simulink model "pd_path_sg"  (R2013b)
settings: Solver=ode45  StartTime=0.0  StopTime=10  RelTol=1e-3
undefined symbols (not defined in the file or in its folder): A, A2, B, C, D, EVAL, i, output_samp_bcoef, PCIN, reg_pk_lim, reg_plim, reg_scale, reg_sr_lim, reg_staclr, reg_txgain, THIS_DATE, W, X, Z
undefined symbols (not defined in the file): lut_address, lut_address_s5, reg_dltap
libraries: xbsIndex_r4 x3819, lut_ram_vhdl x32
(part 2 of 31)

== system pd_path_sg/gmp_model_A ==
  chi : Inport
  x : Inport  Port=2
  c : Inport  Port=3
  Delay1 : xbsIndex_r4/Delay  rst=off  infoeditControl=Selection of Reset will increase slice count due to use of real FFs and instead of SRLs  en=off  latency=1  reg_retiming=off  dbl_ovrd=off  block_type=delay
      settings: infoedit=Hardware notes: A delay line is a chain, each link of which is an SRL16 or SRL32 followed by a flip-flop.
  Delay2 : xbsIndex_r4/Delay  rst=off  infoeditControl=Selection of Reset will increase slice count due to use of real FFs and instead of SRLs  en=off  latency=1  reg_retiming=off  dbl_ovrd=off  block_type=delay
      settings: infoedit=Hardware notes: A delay line is a chain, each link of which is an SRL16 or SRL32 followed by a flip-flop.
  Delay3 : xbsIndex_r4/Delay  rst=off  infoeditControl=Selection of Reset will increase slice count due to use of real FFs and instead of SRLs  en=off  latency=1  reg_retiming=off  dbl_ovrd=off  block_type=delay
      settings: infoedit=Hardware notes: A delay line is a chain, each link of which is an SRL16 or SRL32 followed by a flip-flop.
  Demux : Demux  Outputs=7
  Demux1 : Demux  Outputs=7
  Mux : Mux  Inputs=2
  bit_cut : Subsystem  mask{cut=12, left=17}
  bit_cut1 : Subsystem  mask{cut=12, left=17}
  cmp_mul 0 : Subsystem
  cmp_mul1 : Subsystem
  cmp_mul2 : Subsystem
  cmp_mul3 : Subsystem
  cmp_mul4 : Subsystem
  cmp_mul5 : Subsystem
  cmp_mul6 : Subsystem
  cho : Outport
  y : Outport  Port=2
  wires:
  Demux/1 -> [x0]
  cmp_mul 0/3(pcout_i) -> cmp_mul1/3(pcin_i)
  Mux/1 -> y/1
  x/1 -> Demux/1
  c/1 -> Demux1/1
  cmp_mul 0/4(pcout_q) -> cmp_mul1/4(pcin_q)
  [x0] -> cmp_mul 0/1(x)
  Demux/2 -> [x1]
  [x1] -> cmp_mul1/1(x)
  Demux/3 -> [x2]
  [x2] -> cmp_mul2/1(x)
  Demux/4 -> [x3]
  Demux/5 -> [x4]
  Demux/6 -> [x5]
  Demux/7 -> [x6]
  Demux1/1 -> [c0]
  [c0] -> cmp_mul 0/2(coef)
  [c1] -> cmp_mul1/2(coef)
  Demux1/2 -> [c1]
  [c2] -> cmp_mul2/2(coef)
  Demux1/3 -> [c2]
  Demux1/4 -> [c3]
  Demux1/5 -> [c4]
  Demux1/6 -> [c5]
  Demux1/7 -> [c6]
  Delay1/1 -> Mux/1
  Delay2/1 -> Mux/2
  bit_cut/1(q) -> Delay1/1
  bit_cut1/1(q) -> Delay2/1
  cmp_mul1/3(pcout_i) -> cmp_mul2/3(pcin_i)
  cmp_mul1/4(pcout_q) -> cmp_mul2/4(pcin_q)
  cmp_mul2/3(pcout_i) -> cmp_mul3/3(pcin_i)
  cmp_mul2/4(pcout_q) -> cmp_mul3/4(pcin_q)
  [x3] -> cmp_mul3/1(x)
  [c3] -> cmp_mul3/2(coef)
  cmp_mul3/3(pcout_i) -> cmp_mul4/3(pcin_i)
  cmp_mul3/4(pcout_q) -> cmp_mul4/4(pcin_q)
  [c4] -> cmp_mul4/2(coef)
  [x4] -> cmp_mul4/1(x)
  cmp_mul4/3(pcout_i) -> cmp_mul5/3(pcin_i)
  cmp_mul4/4(pcout_q) -> cmp_mul5/4(pcin_q)
  [c5] -> cmp_mul5/2(coef)
  [x5] -> cmp_mul5/1(x)
  cmp_mul5/3(pcout_i) -> cmp_mul6/3(pcin_i)
  cmp_mul5/4(pcout_q) -> cmp_mul6/4(pcin_q)
  [x6] -> cmp_mul6/1(x)
  [c6] -> cmp_mul6/2(coef)
  cmp_mul6/3(iout) -> bit_cut/1(d)
  cmp_mul6/4(qout) -> bit_cut1/1(d)
  chi/1 -> Delay3/1
  Delay3/1 -> cho/1

== system pd_path_sg/gmp_model_B ==
  chi : Inport
  x : Inport  Port=2
  c : Inport  Port=3
  Delay1 : xbsIndex_r4/Delay  rst=off  infoeditControl=Selection of Reset will increase slice count due to use of real FFs and instead of SRLs  en=off  latency=1  reg_retiming=off  dbl_ovrd=off  block_type=delay
      settings: infoedit=Hardware notes: A delay line is a chain, each link of which is an SRL16 or SRL32 followed by a flip-flop.
  Delay2 : xbsIndex_r4/Delay  rst=off  infoeditControl=Selection of Reset will increase slice count due to use of real FFs and instead of SRLs  en=off  latency=1  reg_retiming=off  dbl_ovrd=off  block_type=delay
      settings: infoedit=Hardware notes: A delay line is a chain, each link of which is an SRL16 or SRL32 followed by a flip-flop.
  Delay3 : xbsIndex_r4/Delay  rst=off  infoeditControl=Selection of Reset will increase slice count due to use of real FFs and instead of SRLs  en=off  latency=1  reg_retiming=off  dbl_ovrd=off  block_type=delay
      settings: infoedit=Hardware notes: A delay line is a chain, each link of which is an SRL16 or SRL32 followed by a flip-flop.
  Demux : Demux  Outputs=7
  Demux1 : Demux  Outputs=7
  Mux : Mux  Inputs=2
  bit_cut : Subsystem  mask{cut=12, left=17}
  bit_cut1 : Subsystem  mask{cut=12, left=17}
  cmp_mul 0 : Subsystem
  cmp_mul1 : Subsystem
  cmp_mul2 : Subsystem
  cmp_mul3 : Subsystem
  cmp_mul4 : Subsystem
  cmp_mul5 : Subsystem
  cmp_mul6 : Subsystem
  cho : Outport
  y : Outport  Port=2
  wires:
  Delay3/1 -> cho/1
  chi/1 -> Delay3/1
  cmp_mul6/4(qout) -> bit_cut1/1(d)
  cmp_mul6/3(iout) -> bit_cut/1(d)
  [c6] -> cmp_mul6/2(coef)
  [x6] -> cmp_mul6/1(x)
  cmp_mul5/4(pcout_q) -> cmp_mul6/4(pcin_q)
  cmp_mul5/3(pcout_i) -> cmp_mul6/3(pcin_i)
  [x5] -> cmp_mul5/1(x)
  [c5] -> cmp_mul5/2(coef)
  cmp_mul4/4(pcout_q) -> cmp_mul5/4(pcin_q)
  cmp_mul4/3(pcout_i) -> cmp_mul5/3(pcin_i)
  [x4] -> cmp_mul4/1(x)
  [c4] -> cmp_mul4/2(coef)
  cmp_mul3/4(pcout_q) -> cmp_mul4/4(pcin_q)
  cmp_mul3/3(pcout_i) -> cmp_mul4/3(pcin_i)
  [c3] -> cmp_mul3/2(coef)
  [x3] -> cmp_mul3/1(x)
  cmp_mul2/4(pcout_q) -> cmp_mul3/4(pcin_q)
  cmp_mul2/3(pcout_i) -> cmp_mul3/3(pcin_i)
  cmp_mul1/4(pcout_q) -> cmp_mul2/4(pcin_q)
  cmp_mul1/3(pcout_i) -> cmp_mul2/3(pcin_i)
  bit_cut1/1(q) -> Delay2/1
  bit_cut/1(q) -> Delay1/1
  Delay2/1 -> Mux/2
  Delay1/1 -> Mux/1
  Demux1/7 -> [c6]
  Demux1/6 -> [c5]
  Demux1/5 -> [c4]
  Demux1/4 -> [c3]
  Demux1/3 -> [c2]
  [c2] -> cmp_mul2/2(coef)
  Demux1/2 -> [c1]
  [c1] -> cmp_mul1/2(coef)
  [c0] -> cmp_mul 0/2(coef)
  Demux1/1 -> [c0]
  Demux/7 -> [x6]
  Demux/6 -> [x5]
  Demux/5 -> [x4]
  Demux/4 -> [x3]
  [x2] -> cmp_mul2/1(x)
  Demux/3 -> [x2]
  [x1] -> cmp_mul1/1(x)
  Demux/2 -> [x1]
  [x0] -> cmp_mul 0/1(x)
  cmp_mul 0/4(pcout_q) -> cmp_mul1/4(pcin_q)
  c/1 -> Demux1/1
  x/1 -> Demux/1
  Mux/1 -> y/1
  cmp_mul 0/3(pcout_i) -> cmp_mul1/3(pcin_i)
  Demux/1 -> [x0]

== system pd_path_sg/input_samp_a ==
  note: nee no delay
  chi : Inport
  sig_valid : Inport  Port=2
  x : Inport  Port=3
  Delay : xbsIndex_r4/Delay  rst=off  infoeditControl=Selection of Reset will increase slice count due to use of real FFs and instead of SRLs  en=off  latency=2  reg_retiming=off  dbl_ovrd=off  block_type=delay
      settings: infoedit=Hardware notes: A delay line is a chain, each link of which is an SRL16 or SRL32 followed by a flip-flop.
  Delay1 : xbsIndex_r4/Delay  rst=off  infoeditControl=Selection of Reset will increase slice count due to use of real FFs and instead of SRLs  en=off  latency=7  reg_retiming=off  dbl_ovrd=off  block_type=delay
      settings: infoedit=Hardware notes: A delay line is a chain, each link of which is an SRL16 or SRL32 followed by a flip-flop.
  Delay2 : xbsIndex_r4/Delay  rst=off  infoeditControl=Selection of Reset will increase slice count due to use of real FFs and instead of SRLs  en=off  latency=2  reg_retiming=off  dbl_ovrd=off  block_type=delay
      settings: infoedit=Hardware notes: A delay line is a chain, each link of which is an SRL16 or SRL32 followed by a flip-flop.
  Demux : Demux  Outputs=2
  Mux : xbsIndex_r4/Mux  inputs=2  en=off  latency=1  precision=Full  arith_type=Unsigned  n_bits=16  bin_pt=14  quantization=Truncate  overflow=Wrap  dbl_ovrd=off  block_type=mux
  Mux1 : Mux  Inputs=2
  input_samp : Subsystem
  muxi : xbsIndex_r4/Mux  inputs=2  en=off  latency=1  precision=Full  arith_type=Unsigned  n_bits=16  bin_pt=14  quantization=Truncate  overflow=Wrap  dbl_ovrd=off  block_type=mux
  muxq : xbsIndex_r4/Mux  inputs=2  en=off  latency=1  precision=Full  arith_type=Unsigned  n_bits=16  bin_pt=14  quantization=Truncate  overflow=Wrap  dbl_ovrd=off  block_type=mux
  cho : Outport
  y : Outport  Port=2
  wires:
  Delay1/1 -> muxi/1, muxq/1
  input_samp/2(interp_seq) -> muxi/3, muxq/2
  input_samp/1(ori_seq) -> muxi/2, muxq/3
  muxi/1 -> Delay2/1
  sig_valid/1 -> Mux/1, Delay1/1
  x/1 -> Demux/1
  Delay/1 -> Mux/2
  Mux/1 -> input_samp/1(In1)
  Demux/1 -> Mux/3
  Demux/2 -> Delay/1
  muxq/1 -> Mux1/2  "yq"
  Delay2/1 -> Mux1/1  "yi"
  Mux1/1 -> y/1
  chi/1 -> cho/1

== system pd_path_sg/input_samp_b ==
  note: nee no delay
  chi : Inport
  sig_valid : Inport  Port=2
  x : Inport  Port=3
  Delay : xbsIndex_r4/Delay  rst=off  infoeditControl=Selection of Reset will increase slice count due to use of real FFs and instead of SRLs  en=off  latency=2  reg_retiming=off  dbl_ovrd=off  block_type=delay
      settings: infoedit=Hardware notes: A delay line is a chain, each link of which is an SRL16 or SRL32 followed by a flip-flop.
  Delay1 : xbsIndex_r4/Delay  rst=off  infoeditControl=Selection of Reset will increase slice count due to use of real FFs and instead of SRLs  en=off  latency=7  reg_retiming=off  dbl_ovrd=off  block_type=delay
      settings: infoedit=Hardware notes: A delay line is a chain, each link of which is an SRL16 or SRL32 followed by a flip-flop.
  Delay2 : xbsIndex_r4/Delay  rst=off  infoeditControl=Selection of Reset will increase slice count due to use of real FFs and instead of SRLs  en=off  latency=2  reg_retiming=off  dbl_ovrd=off  block_type=delay
      settings: infoedit=Hardware notes: A delay line is a chain, each link of which is an SRL16 or SRL32 followed by a flip-flop.
  Demux : Demux  Outputs=2
  Mux : xbsIndex_r4/Mux  inputs=2  en=off  latency=1  precision=Full  arith_type=Unsigned  n_bits=16  bin_pt=14  quantization=Truncate  overflow=Wrap  dbl_ovrd=off  block_type=mux
  Mux1 : Mux  Inputs=2
  input_samp : Subsystem
  muxi : xbsIndex_r4/Mux  inputs=2  en=off  latency=1  precision=Full  arith_type=Unsigned  n_bits=16  bin_pt=14  quantization=Truncate  overflow=Wrap  dbl_ovrd=off  block_type=mux
  muxq : xbsIndex_r4/Mux  inputs=2  en=off  latency=1  precision=Full  arith_type=Unsigned  n_bits=16  bin_pt=14  quantization=Truncate  overflow=Wrap  dbl_ovrd=off  block_type=mux
  cho : Outport
  y : Outport  Port=2
  wires:
  chi/1 -> cho/1
  Mux1/1 -> y/1
  Delay2/1 -> Mux1/1  "yi"
  muxq/1 -> Mux1/2  "yq"
  Demux/2 -> Delay/1
  Demux/1 -> Mux/3
  Mux/1 -> input_samp/1(In1)
  Delay/1 -> Mux/2
  x/1 -> Demux/1
  sig_valid/1 -> Delay1/1, Mux/1
  muxi/1 -> Delay2/1
  input_samp/1(ori_seq) -> muxq/3, muxi/2
  input_samp/2(interp_seq) -> muxq/2, muxi/3
  Delay1/1 -> muxq/1, muxi/1

== system pd_path_sg/insig_source ==
  chnsel : Inport
  chi : Inport  Port=2
  ax : Inport  Port=3
  bx : Inport  Port=4
  Delay : xbsIndex_r4/Delay  rst=off  infoeditControl=Selection of Reset will increase slice count due to use of real FFs and instead of SRLs  en=off  latency=1  reg_retiming=off  dbl_ovrd=off  block_type=delay
      settings: infoedit=Hardware notes: A delay line is a chain, each link of which is an SRL16 or SRL32 followed by a flip-flop.
  Demux1 : Demux  Outputs=2
  Demux2 : Demux  Outputs=2
  Register{,1..3} (4 alike) : xbsIndex_r4/Register  init=0  rst=off  en=on  dbl_ovrd=off  block_type=register
  Relational : xbsIndex_r4/Relational  mode=a=b  op_type=Bool  en=off  latency=0  dbl_ovrd=off  block_type=relational
  srcval : Outport
  asrci : Outport  Port=2
  asrcq : Outport  Port=3
  bsrci : Outport  Port=4
  bsrcq : Outport  Port=5
  wires:
  ax/1 -> Demux2/1
  bx/1 -> Demux1/1
  chnsel/1 -> Relational/1
  chi/1 -> Relational/2
  Demux2/1 -> Register/1
  Delay/1 -> srcval/1
  Demux2/2 -> Register1/1
  Demux1/1 -> Register2/1
  Demux1/2 -> Register3/1
  Relational/1 -> Delay/1, Register1/2, Register2/2, Register3/2, Register/2
  Register/1 -> asrci/1
  Register1/1 -> asrcq/1
  Register2/1 -> bsrci/1
  Register3/1 -> bsrcq/1

== system pd_path_sg/insig_source1 ==
  chnsel : Inport
  chi : Inport  Port=2
  ax : Inport  Port=3
  bx : Inport  Port=4
  Delay : xbsIndex_r4/Delay  rst=off  infoeditControl=Selection of Reset will increase slice count due to use of real FFs and instead of SRLs  en=off  latency=1  reg_retiming=off  dbl_ovrd=off  block_type=delay
      settings: infoedit=Hardware notes: A delay line is a chain, each link of which is an SRL16 or SRL32 followed by a flip-flop.
  Demux1 : Demux  Outputs=2
  Demux2 : Demux  Outputs=2
  Register{,1..3} (4 alike) : xbsIndex_r4/Register  init=0  rst=off  en=on  dbl_ovrd=off  block_type=register
  Relational : xbsIndex_r4/Relational  mode=a=b  op_type=Bool  en=off  latency=0  dbl_ovrd=off  block_type=relational
  Slice{1..4} (4 alike) : xbsIndex_r4/Slice  nbits=16  boolean_output=off  mode=Lower Bit Location + Width  bit1=0  base1=MSB of Input  bit0=0  base0=LSB of Input  dbl_ovrd=off  block_type=slice
  srcval : Outport
  asrci : Outport  Port=2
  asrcq : Outport  Port=3
  bsrci : Outport  Port=4
  bsrcq : Outport  Port=5
  wires:
  Register3/1 -> bsrcq/1
  Register2/1 -> bsrci/1
  Register1/1 -> asrcq/1
  Register/1 -> asrci/1
  Relational/1 -> Register/2, Register3/2, Register2/2, Register1/2, Delay/1
  Demux1/2 -> Slice4/1
  Demux1/1 -> Slice3/1
  Demux2/2 -> Slice1/1
  Delay/1 -> srcval/1
  Demux2/1 -> Slice2/1
  chi/1 -> Relational/2
  chnsel/1 -> Relational/1
  bx/1 -> Demux1/1
  ax/1 -> Demux2/1
  Slice2/1 -> Register/1
  Slice1/1 -> Register1/1
  Slice3/1 -> Register2/1
  Slice4/1 -> Register3/1

== system pd_path_sg/iq_delay ==
  x : Inport
  Delay : xbsIndex_r4/Delay  rst=off  infoeditControl=Selection of Reset will increase slice count due to use of real FFs and instead of SRLs  en=off  latency=clocks  reg_retiming=off  dbl_ovrd=off  block_type=delay
      settings: infoedit=Hardware notes: A delay line is a chain, each link of which is an SRL16 or SRL32 followed by a flip-flop.
  Delay1 : xbsIndex_r4/Delay  rst=off  infoeditControl=Selection of Reset will increase slice count due to use of real FFs and instead of SRLs  en=off  latency=clocks  reg_retiming=off  dbl_ovrd=off  block_type=delay
      settings: infoedit=Hardware notes: A delay line is a chain, each link of which is an SRL16 or SRL32 followed by a flip-flop.
  Demux : Demux  Outputs=2
  Mux : Mux  Inputs=2
  y : Outport
  wires:
  Delay1/1 -> Mux/2
  Demux/2 -> Delay1/1
  Demux/1 -> Delay/1
  Mux/1 -> y/1
  Delay/1 -> Mux/1
  x/1 -> Demux/1

== system pd_path_sg/iq_delay1 ==
  x : Inport
  Delay : xbsIndex_r4/Delay  rst=off  infoeditControl=Selection of Reset will increase slice count due to use of real FFs and instead of SRLs  en=off  latency=clocks  reg_retiming=off  dbl_ovrd=off  block_type=delay
      settings: infoedit=Hardware notes: A delay line is a chain, each link of which is an SRL16 or SRL32 followed by a flip-flop.
  Delay1 : xbsIndex_r4/Delay  rst=off  infoeditControl=Selection of Reset will increase slice count due to use of real FFs and instead of SRLs  en=off  latency=clocks  reg_retiming=off  dbl_ovrd=off  block_type=delay
      settings: infoedit=Hardware notes: A delay line is a chain, each link of which is an SRL16 or SRL32 followed by a flip-flop.
  Demux : Demux  Outputs=2
  Mux : Mux  Inputs=2
  y : Outport
  wires:
  x/1 -> Demux/1
  Delay/1 -> Mux/1
  Mux/1 -> y/1
  Demux/1 -> Delay/1
  Demux/2 -> Delay1/1
  Delay1/1 -> Mux/2

== system pd_path_sg/other_regs ==
  per : Inport
  Bus Selector : BusSelector  OutputSignals=addr,din,we
  Delay : xbsIndex_r4/Delay  rst=off  infoeditControl=Selection of Reset will increase slice count due to use of real FFs and instead of SRLs  en=off  latency=1  reg_retiming=off  dbl_ovrd=off  block_type=delay
  Delay1 : xbsIndex_r4/Delay  rst=off  infoeditControl=Selection of Reset will increase slice count due to use of real FFs and instead of SRLs  en=off  latency=1  reg_retiming=off  dbl_ovrd=off  block_type=delay
  Delay2 : xbsIndex_r4/Delay  rst=off  infoeditControl=Selection of Reset will increase slice count due to use of real FFs and instead of SRLs  en=off  latency=1  reg_retiming=off  dbl_ovrd=off  block_type=delay
  perbus_reg : Subsystem
  bandsel : Outport
  lut_active : Outport  Port=2
  wires:
  Bus Selector/2 -> Delay1/1  "<din>"
  Bus Selector/1 -> Delay/1  "<addr>"
  Bus Selector/3 -> Delay2/1  "<we>"
  per/1 -> Bus Selector/1
  perbus_reg/2(lut_active) -> lut_active/1
  perbus_reg/1(band) -> bandsel/1
  Delay/1 -> perbus_reg/1(addr)
  Delay1/1 -> perbus_reg/2(din)
  Delay2/1 -> perbus_reg/3(we)

== system pd_path_sg/output_gainA ==
  chi : Inport
  x : Inport  Port=2
  gain0 : Inport  Port=3
  gain1 : Inport  Port=4
  ext_gain0 : Inport  Port=5
  ext_gain1 : Inport  Port=6
  Constant1 : xbsIndex_r4/Constant  const=0  gui_display_data_type=Fixed-point  arith_type=Unsigned  n_bits=16  bin_pt=0  preci_type=Single  exp_width=8  frac_width=24  explicit_period=off  period=1  equ=P=C  opselect=C  inp2=PCIN>>17  opr=+  inp1=P  carry=CIN  dbl_ovrd=off  block_type=constant
  Constant2 : xbsIndex_r4/Constant  const=0  gui_display_data_type=Fixed-point  arith_type=Unsigned  n_bits=16  bin_pt=0  preci_type=Single  exp_width=8  frac_width=24  explicit_period=off  period=1  equ=P=C  opselect=C  inp2=PCIN>>17  opr=+  inp1=P  carry=CIN  dbl_ovrd=off  block_type=constant
  Convert : xbsIndex_r4/Convert  gui_display_data_type=Fixed-point  arith_type="Signed  (2's comp)"  n_bits=30  bin_pt=0  float_type=Single  exp_bits=8  fraction_bits=24  quantization=Truncate  overflow=Wrap  en=off  latency=0  pipeline=off  dbl_ovrd=off  block_type=convert
  Convert1 : xbsIndex_r4/Convert  gui_display_data_type=Fixed-point  arith_type="Signed  (2's comp)"  n_bits=18  bin_pt=0  float_type=Single  exp_bits=8  fraction_bits=24  quantization=Truncate  overflow=Wrap  en=off  latency=0  pipeline=off  dbl_ovrd=off  block_type=convert
  Convert2 : xbsIndex_r4/Convert  gui_display_data_type=Fixed-point  arith_type="Signed  (2's comp)"  n_bits=30  bin_pt=0  float_type=Single  exp_bits=8  fraction_bits=24  quantization=Truncate  overflow=Wrap  en=off  latency=0  pipeline=off  dbl_ovrd=off  block_type=convert
  Convert3 : xbsIndex_r4/Convert  gui_display_data_type=Fixed-point  arith_type="Signed  (2's comp)"  n_bits=18  bin_pt=0  float_type=Single  exp_bits=8  fraction_bits=24  quantization=Truncate  overflow=Wrap  en=off  latency=0  pipeline=off  dbl_ovrd=off  block_type=convert
  "DSP48E2 " : xbsIndex_r4/DSP48E2   use_a=Direct from A Port  use_b=Direct from B Port  addsub_mode=ONE48  xl_useadderonly=off  xl_dynamicmult=off  preaddinsel=A  amultsel=A  bmultsel=B  enable_d=off  reset_preg=off  auto_reset_pr=RESET  pattern_from_creg=1  pattern='000000000000'  mask_from_creg=1  pattern_mask='000000000000'  rnd='000000000000'  widexor=off  xormode=1  use_op=on  use_creg=off  rst_all=off  en_all=off  use_pcin=off  use_carrycascin=off  use_multsignin=off  use_carryout=off  use_patterndetect=off  use_patternbdetect=off  use_overflow=off  use_underflow=off  use_acout=off  use_bcout=off  use_pcout=off  use_multsignout=off  use_carrycascout=off  pipeline_a=1  pipeline_b=1  pipeline_acout=1  pipeline_bcout=1  pipeline_c=on  pipeline_p=on  pipeline_mult=on  pipeline_opmode=on  pipeline_alumode=on  pipeline_carryin=on  pipeline_carryinsel=on  dreg=off  adreg=off  register_inmode=off  rst_a=off  rst_b=off  rst_c=off  rst_mult=off  rst_p=off  rst_carry_in=off  rst_alumode=off  rst_ctrl=off  reset_port_d=off  reset_port_inmode=off  en_a1=off  en_a2=off  en_b1=off  en_b2=off  en_c=off  en_mult=off  en_p=off  en_carry_in=off  en_alumode=off  en_multcarryin=off  en_ctrl=off  enable_port_regd=off  enable_port_regad=off  enable_port_reginmode=off  alumode_inverted=off  alumode_inverted_value='0000'  is_carryin_inverted=off  inmode_inverted=off  inmode_inverted_value='00000'  opmode_inverted=off  opmode_inverted_value='000000000'  is_rstallcarryin_inverted=off  is_rstalumode_inverted=off  is_rsta_inverted=off  is_rstb_inverted=off  is_rstc_inverted=off  is_rstd_inverted=off  is_rstctrl_inverted=off  is_rstinmode_inverted=off  is_rstm_inverted=off  is_rstp_inverted=off  use_synth_model=off  is_clk_inverted=false  block_type=dsp48e2
  DSP48E2 1 : xbsIndex_r4/DSP48E2   use_a=Direct from A Port  use_b=Direct from B Port  addsub_mode=ONE48  xl_useadderonly=off  xl_dynamicmult=off  preaddinsel=A  amultsel=A  bmultsel=B  enable_d=off  reset_preg=off  auto_reset_pr=RESET  pattern_from_creg=1  pattern='000000000000'  mask_from_creg=1  pattern_mask='000000000000'  rnd='000000000000'  widexor=off  xormode=1  use_op=on  use_creg=off  rst_all=off  en_all=off  use_pcin=off  use_carrycascin=off  use_multsignin=off  use_carryout=off  use_patterndetect=off  use_patternbdetect=off  use_overflow=off  use_underflow=off  use_acout=off  use_bcout=off  use_pcout=off  use_multsignout=off  use_carrycascout=off  pipeline_a=1  pipeline_b=1  pipeline_acout=1  pipeline_bcout=1  pipeline_c=on  pipeline_p=on  pipeline_mult=on  pipeline_opmode=on  pipeline_alumode=on  pipeline_carryin=on  pipeline_carryinsel=on  dreg=off  adreg=off  register_inmode=off  rst_a=off  rst_b=off  rst_c=off  rst_mult=off  rst_p=off  rst_carry_in=off  rst_alumode=off  rst_ctrl=off  reset_port_d=off  reset_port_inmode=off  en_a1=off  en_a2=off  en_b1=off  en_b2=off  en_c=off  en_mult=off  en_p=off  en_carry_in=off  en_alumode=off  en_multcarryin=off  en_ctrl=off  enable_port_regd=off  enable_port_regad=off  enable_port_reginmode=off  alumode_inverted=off  alumode_inverted_value='0000'  is_carryin_inverted=off  inmode_inverted=off  inmode_inverted_value='00000'  opmode_inverted=off  opmode_inverted_value='000000000'  is_rstallcarryin_inverted=off  is_rstalumode_inverted=off  is_rsta_inverted=off  is_rstb_inverted=off  is_rstc_inverted=off  is_rstd_inverted=off  is_rstctrl_inverted=off  is_rstinmode_inverted=off  is_rstm_inverted=off  is_rstp_inverted=off  use_synth_model=off  is_clk_inverted=false  block_type=dsp48e2
  Delay1 : xbsIndex_r4/Delay  rst=off  infoeditControl=Selection of Reset will increase slice count due to use of real FFs and instead of SRLs  en=off  latency=1  reg_retiming=off  dbl_ovrd=off  block_type=delay
  Delay3 : xbsIndex_r4/Delay  rst=off  infoeditControl=Selection of Reset will increase slice count due to use of real FFs and instead of SRLs  en=off  latency=1  reg_retiming=off  dbl_ovrd=off  block_type=delay
  Demux : Demux  Outputs=2
  Mux : Mux  Inputs=2
  Mux0 : xbsIndex_r4/Mux  inputs=2  en=off  latency=1  precision=Full  arith_type=Unsigned  n_bits=16  bin_pt=14  quantization=Truncate  overflow=Wrap  dbl_ovrd=off  block_type=mux
  Mux1 : xbsIndex_r4/Mux  inputs=2  en=off  latency=1  precision=Full  arith_type=Unsigned  n_bits=16  bin_pt=14  quantization=Truncate  overflow=Wrap  dbl_ovrd=off  block_type=mux
  Mux2 : xbsIndex_r4/Mux  inputs=2  en=off  latency=1  precision=Full  arith_type=Unsigned  n_bits=16  bin_pt=14  quantization=Truncate  overflow=Wrap  dbl_ovrd=off  block_type=mux
  Opmode : xbsIndex_r4/Opmode  device=DSP48E2  equ=P=(A*B)+RND  operation=Custom  inmode_0_3=D+A2  inmode_1_3=A*B  preaddinsel=A  amultsel=A  bmultsel=B  inmode_0=A2  inmode_4=B2  logicinstr=X + W + Z  z_mux=0  xy_mux=A*B  w_mux=RND  carry=0  dbl_ovrd=off  operand=+  x_mux=P  block_type=opmode
  Opmode1 : xbsIndex_r4/Opmode  device=DSP48E2  equ=P=(A*B)+RND  operation=Custom  inmode_0_3=D+A2  inmode_1_3=A*B  preaddinsel=A  amultsel=A  bmultsel=B  inmode_0=A2  inmode_4=B2  logicinstr=X + W + Z  z_mux=0  xy_mux=A*B  w_mux=RND  carry=0  dbl_ovrd=off  operand=+  x_mux=P  block_type=opmode
  Reinterpret1 : xbsIndex_r4/Reinterpret  force_arith_type=on  arith_type="Signed  (2's comp)"  force_bin_pt=off  bin_pt=0  block_type=reinterpret
  Reinterpret4 : xbsIndex_r4/Reinterpret  force_arith_type=on  arith_type="Signed  (2's comp)"  force_bin_pt=off  bin_pt=0  block_type=reinterpret
  Relational : xbsIndex_r4/Relational  mode=a=b  op_type=Bool  en=off  latency=0  dbl_ovrd=off  block_type=relational
  Relational1 : xbsIndex_r4/Relational  mode=a=b  op_type=Bool  en=off  latency=0  dbl_ovrd=off  block_type=relational
  Slice1 : xbsIndex_r4/Slice  nbits=17  boolean_output=off  mode=Lower Bit Location + Width  bit1=0  base1=MSB of Input  bit0=14  base0=LSB of Input  dbl_ovrd=off  block_type=slice
  Slice2 : xbsIndex_r4/Slice  nbits=17  boolean_output=off  mode=Lower Bit Location + Width  bit1=0  base1=MSB of Input  bit0=14  base0=LSB of Input  dbl_ovrd=off  block_type=slice
  copied : xbsIndex_r4/Mux  inputs=2  en=off  latency=1  precision=Full  arith_type=Unsigned  n_bits=16  bin_pt=14  quantization=Truncate  overflow=Wrap  dbl_ovrd=off  block_type=mux
  preset_1clock : xbsIndex_r4/Delay  rst=off  infoeditControl=Selection of Reset will increase slice count due to use of real FFs and instead of SRLs  en=off  latency=1  reg_retiming=off  dbl_ovrd=off  block_type=delay
  preset_1clock1 : xbsIndex_r4/Delay  rst=off  infoeditControl=Selection of Reset will increase slice count due to use of real FFs and instead of SRLs  en=off  latency=4  reg_retiming=off  dbl_ovrd=off  block_type=delay
      settings: infoedit=Hardware notes: A delay line is a chain, each link of which is an SRL16 or SRL32 followed by a flip-flop.
  cho : Outport
  y : Outport  Port=2
  wires:
  ext_gain0/1 -> Mux0/2, Relational/1
  Constant1/1 -> Relational/2
  Relational/1 -> Mux0/1
  gain0/1 -> Mux0/3
  ext_gain1/1 -> Relational1/1, Mux1/2
  Constant2/1 -> Relational1/2
  Relational1/1 -> Mux1/1
  gain1/1 -> Mux1/3
  Mux0/1 -> Mux2/2, copied/2
  chi/1 -> preset_1clock1/1, preset_1clock/1
  Mux1/1 -> Mux2/3, copied/3
  Opmode/1 -> "DSP48E2 "/3
  Convert1/1 -> "DSP48E2 "/2
  Convert/1 -> "DSP48E2 "/1
  Mux2/1 -> Convert1/1
  x/1 -> Demux/1
  Convert3/1 -> DSP48E2 1/2
  Convert2/1 -> DSP48E2 1/1
  copied/1 -> Convert3/1
  Demux/1 -> Convert/1
  Demux/2 -> Convert2/1
  Slice2/1 -> Delay3/1
  Mux/1 -> y/1
  Delay3/1 -> Reinterpret4/1
  Slice1/1 -> Delay1/1
  DSP48E2 1/1 -> Slice1/1
  "DSP48E2 "/1 -> Slice2/1
  Delay1/1 -> Reinterpret1/1
  Reinterpret4/1 -> Mux/1
  Reinterpret1/1 -> Mux/2
  Opmode1/1 -> DSP48E2 1/3
  preset_1clock/1 -> copied/1, Mux2/1
  preset_1clock1/1 -> cho/1

== system pd_path_sg/output_gainB ==
  chi : Inport
  x : Inport  Port=2
  gain0 : Inport  Port=3
  gain1 : Inport  Port=4
  ext_gain0 : Inport  Port=5
  ext_gain1 : Inport  Port=6
  Constant1 : xbsIndex_r4/Constant  const=0  gui_display_data_type=Fixed-point  arith_type=Unsigned  n_bits=16  bin_pt=0  preci_type=Single  exp_width=8  frac_width=24  explicit_period=off  period=1  equ=P=C  opselect=C  inp2=PCIN>>17  opr=+  inp1=P  carry=CIN  dbl_ovrd=off  block_type=constant
  Constant2 : xbsIndex_r4/Constant  const=0  gui_display_data_type=Fixed-point  arith_type=Unsigned  n_bits=16  bin_pt=0  preci_type=Single  exp_width=8  frac_width=24  explicit_period=off  period=1  equ=P=C  opselect=C  inp2=PCIN>>17  opr=+  inp1=P  carry=CIN  dbl_ovrd=off  block_type=constant
  Convert : xbsIndex_r4/Convert  gui_display_data_type=Fixed-point  arith_type="Signed  (2's comp)"  n_bits=30  bin_pt=0  float_type=Single  exp_bits=8  fraction_bits=24  quantization=Truncate  overflow=Wrap  en=off  latency=0  pipeline=off  dbl_ovrd=off  block_type=convert
  Convert1 : xbsIndex_r4/Convert  gui_display_data_type=Fixed-point  arith_type="Signed  (2's comp)"  n_bits=18  bin_pt=0  float_type=Single  exp_bits=8  fraction_bits=24  quantization=Truncate  overflow=Wrap  en=off  latency=0  pipeline=off  dbl_ovrd=off  block_type=convert
  Convert2 : xbsIndex_r4/Convert  gui_display_data_type=Fixed-point  arith_type="Signed  (2's comp)"  n_bits=30  bin_pt=0  float_type=Single  exp_bits=8  fraction_bits=24  quantization=Truncate  overflow=Wrap  en=off  latency=0  pipeline=off  dbl_ovrd=off  block_type=convert
  Convert3 : xbsIndex_r4/Convert  gui_display_data_type=Fixed-point  arith_type="Signed  (2's comp)"  n_bits=18  bin_pt=0  float_type=Single  exp_bits=8  fraction_bits=24  quantization=Truncate  overflow=Wrap  en=off  latency=0  pipeline=off  dbl_ovrd=off  block_type=convert
  "DSP48E2 " : xbsIndex_r4/DSP48E2   use_a=Direct from A Port  use_b=Direct from B Port  addsub_mode=ONE48  xl_useadderonly=off  xl_dynamicmult=off  preaddinsel=A  amultsel=A  bmultsel=B  enable_d=off  reset_preg=off  auto_reset_pr=RESET  pattern_from_creg=1  pattern='000000000000'  mask_from_creg=1  pattern_mask='000000000000'  rnd='000000000000'  widexor=off  xormode=1  use_op=on  use_creg=off  rst_all=off  en_all=off  use_pcin=off  use_carrycascin=off  use_multsignin=off  use_carryout=off  use_patterndetect=off  use_patternbdetect=off  use_overflow=off  use_underflow=off  use_acout=off  use_bcout=off  use_pcout=off  use_multsignout=off  use_carrycascout=off  pipeline_a=1  pipeline_b=1  pipeline_acout=1  pipeline_bcout=1  pipeline_c=on  pipeline_p=on  pipeline_mult=on  pipeline_opmode=on  pipeline_alumode=on  pipeline_carryin=on  pipeline_carryinsel=on  dreg=off  adreg=off  register_inmode=off  rst_a=off  rst_b=off  rst_c=off  rst_mult=off  rst_p=off  rst_carry_in=off  rst_alumode=off  rst_ctrl=off  reset_port_d=off  reset_port_inmode=off  en_a1=off  en_a2=off  en_b1=off  en_b2=off  en_c=off  en_mult=off  en_p=off  en_carry_in=off  en_alumode=off  en_multcarryin=off  en_ctrl=off  enable_port_regd=off  enable_port_regad=off  enable_port_reginmode=off  alumode_inverted=off  alumode_inverted_value='0000'  is_carryin_inverted=off  inmode_inverted=off  inmode_inverted_value='00000'  opmode_inverted=off  opmode_inverted_value='000000000'  is_rstallcarryin_inverted=off  is_rstalumode_inverted=off  is_rsta_inverted=off  is_rstb_inverted=off  is_rstc_inverted=off  is_rstd_inverted=off  is_rstctrl_inverted=off  is_rstinmode_inverted=off  is_rstm_inverted=off  is_rstp_inverted=off  use_synth_model=off  is_clk_inverted=false  block_type=dsp48e2
  DSP48E2 1 : xbsIndex_r4/DSP48E2   use_a=Direct from A Port  use_b=Direct from B Port  addsub_mode=ONE48  xl_useadderonly=off  xl_dynamicmult=off  preaddinsel=A  amultsel=A  bmultsel=B  enable_d=off  reset_preg=off  auto_reset_pr=RESET  pattern_from_creg=1  pattern='000000000000'  mask_from_creg=1  pattern_mask='000000000000'  rnd='000000000000'  widexor=off  xormode=1  use_op=on  use_creg=off  rst_all=off  en_all=off  use_pcin=off  use_carrycascin=off  use_multsignin=off  use_carryout=off  use_patterndetect=off  use_patternbdetect=off  use_overflow=off  use_underflow=off  use_acout=off  use_bcout=off  use_pcout=off  use_multsignout=off  use_carrycascout=off  pipeline_a=1  pipeline_b=1  pipeline_acout=1  pipeline_bcout=1  pipeline_c=on  pipeline_p=on  pipeline_mult=on  pipeline_opmode=on  pipeline_alumode=on  pipeline_carryin=on  pipeline_carryinsel=on  dreg=off  adreg=off  register_inmode=off  rst_a=off  rst_b=off  rst_c=off  rst_mult=off  rst_p=off  rst_carry_in=off  rst_alumode=off  rst_ctrl=off  reset_port_d=off  reset_port_inmode=off  en_a1=off  en_a2=off  en_b1=off  en_b2=off  en_c=off  en_mult=off  en_p=off  en_carry_in=off  en_alumode=off  en_multcarryin=off  en_ctrl=off  enable_port_regd=off  enable_port_regad=off  enable_port_reginmode=off  alumode_inverted=off  alumode_inverted_value='0000'  is_carryin_inverted=off  inmode_inverted=off  inmode_inverted_value='00000'  opmode_inverted=off  opmode_inverted_value='000000000'  is_rstallcarryin_inverted=off  is_rstalumode_inverted=off  is_rsta_inverted=off  is_rstb_inverted=off  is_rstc_inverted=off  is_rstd_inverted=off  is_rstctrl_inverted=off  is_rstinmode_inverted=off  is_rstm_inverted=off  is_rstp_inverted=off  use_synth_model=off  is_clk_inverted=false  block_type=dsp48e2
  Delay1 : xbsIndex_r4/Delay  rst=off  infoeditControl=Selection of Reset will increase slice count due to use of real FFs and instead of SRLs  en=off  latency=1  reg_retiming=off  dbl_ovrd=off  block_type=delay
  Delay3 : xbsIndex_r4/Delay  rst=off  infoeditControl=Selection of Reset will increase slice count due to use of real FFs and instead of SRLs  en=off  latency=1  reg_retiming=off  dbl_ovrd=off  block_type=delay
  Demux : Demux  Outputs=2
  Mux : Mux  Inputs=2
  Mux0 : xbsIndex_r4/Mux  inputs=2  en=off  latency=1  precision=Full  arith_type=Unsigned  n_bits=16  bin_pt=14  quantization=Truncate  overflow=Wrap  dbl_ovrd=off  block_type=mux
  Mux1 : xbsIndex_r4/Mux  inputs=2  en=off  latency=1  precision=Full  arith_type=Unsigned  n_bits=16  bin_pt=14  quantization=Truncate  overflow=Wrap  dbl_ovrd=off  block_type=mux
  Mux2 : xbsIndex_r4/Mux  inputs=2  en=off  latency=1  precision=Full  arith_type=Unsigned  n_bits=16  bin_pt=14  quantization=Truncate  overflow=Wrap  dbl_ovrd=off  block_type=mux
  Opmode : xbsIndex_r4/Opmode  device=DSP48E2  equ=P=(A*B)+RND  operation=Custom  inmode_0_3=D+A2  inmode_1_3=A*B  preaddinsel=A  amultsel=A  bmultsel=B  inmode_0=A2  inmode_4=B2  logicinstr=X + W + Z  z_mux=0  xy_mux=A*B  w_mux=RND  carry=0  dbl_ovrd=off  operand=+  x_mux=P  block_type=opmode
  Opmode1 : xbsIndex_r4/Opmode  device=DSP48E2  equ=P=(A*B)+RND  operation=Custom  inmode_0_3=D+A2  inmode_1_3=A*B  preaddinsel=A  amultsel=A  bmultsel=B  inmode_0=A2  inmode_4=B2  logicinstr=X + W + Z  z_mux=0  xy_mux=A*B  w_mux=RND  carry=0  dbl_ovrd=off  operand=+  x_mux=P  block_type=opmode
  Reinterpret1 : xbsIndex_r4/Reinterpret  force_arith_type=on  arith_type="Signed  (2's comp)"  force_bin_pt=off  bin_pt=0  block_type=reinterpret
  Reinterpret4 : xbsIndex_r4/Reinterpret  force_arith_type=on  arith_type="Signed  (2's comp)"  force_bin_pt=off  bin_pt=0  block_type=reinterpret
  Relational : xbsIndex_r4/Relational  mode=a=b  op_type=Bool  en=off  latency=0  dbl_ovrd=off  block_type=relational
  Relational1 : xbsIndex_r4/Relational  mode=a=b  op_type=Bool  en=off  latency=0  dbl_ovrd=off  block_type=relational
  Slice1 : xbsIndex_r4/Slice  nbits=17  boolean_output=off  mode=Lower Bit Location + Width  bit1=0  base1=MSB of Input  bit0=14  base0=LSB of Input  dbl_ovrd=off  block_type=slice
  Slice2 : xbsIndex_r4/Slice  nbits=17  boolean_output=off  mode=Lower Bit Location + Width  bit1=0  base1=MSB of Input  bit0=14  base0=LSB of Input  dbl_ovrd=off  block_type=slice
  copied : xbsIndex_r4/Mux  inputs=2  en=off  latency=1  precision=Full  arith_type=Unsigned  n_bits=16  bin_pt=14  quantization=Truncate  overflow=Wrap  dbl_ovrd=off  block_type=mux
  preset_1clock : xbsIndex_r4/Delay  rst=off  infoeditControl=Selection of Reset will increase slice count due to use of real FFs and instead of SRLs  en=off  latency=1  reg_retiming=off  dbl_ovrd=off  block_type=delay
  preset_1clock1 : xbsIndex_r4/Delay  rst=off  infoeditControl=Selection of Reset will increase slice count due to use of real FFs and instead of SRLs  en=off  latency=4  reg_retiming=off  dbl_ovrd=off  block_type=delay
      settings: infoedit=Hardware notes: A delay line is a chain, each link of which is an SRL16 or SRL32 followed by a flip-flop.
  cho : Outport
  y : Outport  Port=2
  wires:
  preset_1clock1/1 -> cho/1
  preset_1clock/1 -> Mux2/1, copied/1
  Opmode1/1 -> DSP48E2 1/3
  Reinterpret1/1 -> Mux/2
  Reinterpret4/1 -> Mux/1
  Delay1/1 -> Reinterpret1/1
  "DSP48E2 "/1 -> Slice2/1
  DSP48E2 1/1 -> Slice1/1
  Slice1/1 -> Delay1/1
  Delay3/1 -> Reinterpret4/1
  Mux/1 -> y/1
  Slice2/1 -> Delay3/1
  Demux/2 -> Convert2/1
  Demux/1 -> Convert/1
  copied/1 -> Convert3/1
  Convert2/1 -> DSP48E2 1/1
  Convert3/1 -> DSP48E2 1/2
  x/1 -> Demux/1
  Mux2/1 -> Convert1/1
  Convert/1 -> "DSP48E2 "/1
  Convert1/1 -> "DSP48E2 "/2
  Opmode/1 -> "DSP48E2 "/3
  Mux1/1 -> copied/3, Mux2/3
  chi/1 -> preset_1clock/1, preset_1clock1/1
  Mux0/1 -> copied/2, Mux2/2
  gain1/1 -> Mux1/3
  Relational1/1 -> Mux1/1
  Constant2/1 -> Relational1/2
  ext_gain1/1 -> Mux1/2, Relational1/1
  gain0/1 -> Mux0/3
  Relational/1 -> Mux0/1
  Constant1/1 -> Relational/2
  ext_gain0/1 -> Relational/1, Mux0/2

== system pd_path_sg/output_sw_A ==
  chi : Inport
  x : Inport  Port=2
  d : Inport  Port=3
  perbus : Inport  Port=4
  chnsel : Inport  Port=5
  rst : Inport  Port=6
  Demux1 : Demux  Outputs=2
  Demux2 : Demux  Outputs=2
  add_switch : Subsystem  mask{delaytaps=3}
  ch_split : Subsystem
  config_regs0 : Subsystem
  config_regs1 : Subsystem
  detect_i : Subsystem
  detect_q : Subsystem
  on_status : Subsystem
  cho : Outport
  y : Outport  Port=2
  gain0 : Outport  Port=3
  gain1 : Outport  Port=4
  pk_status : Outport  Port=5
  sr_status : Outport  Port=6
  wires:
  perbus/1 -> ch_split/1(per)
  chnsel/1 -> on_status/10(chnsel), ch_split/2(chnsel)
  ch_split/1(per0) -> config_regs0/1(per)
  x/1 -> add_switch/2(x), Demux1/1
  d/1 -> add_switch/3(d), Demux2/1
  Demux1/1 -> detect_i/2(x)
  Demux2/1 -> detect_i/3(d)
  config_regs0/1(sr_lim) -> [sr0]
  config_regs0/2(pk_lim) -> [pk0]
  chi/1 -> add_switch/1(chi), detect_q/1(chi), detect_i/1(chi)
  [pk0] -> detect_i/4(pk0)
  [pk1] -> detect_i/5(pk1)
  [sr0] -> detect_i/6(sr0)
  [sr1] -> detect_i/7(sr1)
  [pk0] -> detect_q/4(pk0)
  [pk1] -> detect_q/5(pk1)
  [sr0] -> detect_q/6(sr0)
  [sr1] -> detect_q/7(sr1)
  Demux1/2 -> detect_q/2(x)
  Demux2/2 -> detect_q/3(d)
  detect_i/1(cho) -> on_status/1(chi)
  detect_i/2(pk_alarm) -> on_status/2(pki_alarm)
  detect_i/3(sr_alarm) -> on_status/3(sri_alarm)
  detect_q/2(pk_alarm) -> on_status/4(pkq_alarm)
  detect_q/3(sr_alarm) -> on_status/5(srq_alarm)
  on_status/3(sw0) -> [sw0]
  on_status/4(sw1) -> [sw1]
  add_switch/2(y) -> y/1
  config_regs0/4(pd_on) -> [on0]
  config_regs1/2(pk_lim) -> [pk1]
  config_regs1/3(alarm_clr) -> [clr1]
  config_regs1/4(pd_on) -> [on1]
  ch_split/2(per1) -> config_regs1/1(per)
  [clr0] -> on_status/6(clr0)
  [clr1] -> on_status/7(clr1)
  [on0] -> on_status/8(on0)
  [on1] -> on_status/9(on1)
  [sw0] -> add_switch/4(on0)
  [sw1] -> add_switch/5(on1)
  config_regs0/5(tx_gain) -> gain0/1
  config_regs1/5(tx_gain) -> gain1/1
  rst/1 -> config_regs0/2(rst), config_regs1/2(rst)
  on_status/1(pk_status) -> pk_status/1
  on_status/2(sr_status) -> sr_status/1
  add_switch/1(cho) -> cho/1
  config_regs1/1(sr_lim) -> [sr1]
  config_regs0/3(alarm_clr) -> [clr0]

== system pd_path_sg/output_sw_B ==
  chi : Inport
  x : Inport  Port=2
  d : Inport  Port=3
  perbus : Inport  Port=4
  chnsel : Inport  Port=5
  rst : Inport  Port=6
  Demux1 : Demux  Outputs=2
  Demux2 : Demux  Outputs=2
  add_switch : Subsystem  mask{delaytaps=3}
  ch_split : Subsystem
  config_regs0 : Subsystem
  config_regs1 : Subsystem
  detect_i : Subsystem
  detect_q : Subsystem
  on_status : Subsystem
  cho : Outport
  y : Outport  Port=2
  gain0 : Outport  Port=3
  gain1 : Outport  Port=4
  pk_status : Outport  Port=5
  sr_status : Outport  Port=6
  wires:
  config_regs0/3(alarm_clr) -> [clr0]
  config_regs1/1(sr_lim) -> [sr1]
  add_switch/1(cho) -> cho/1
  on_status/2(sr_status) -> sr_status/1
  on_status/1(pk_status) -> pk_status/1
  rst/1 -> config_regs1/2(rst), config_regs0/2(rst)
  config_regs1/5(tx_gain) -> gain1/1
  config_regs0/5(tx_gain) -> gain0/1
  [sw1] -> add_switch/5(on1)
  [sw0] -> add_switch/4(on0)
  [on1] -> on_status/9(on1)
  [on0] -> on_status/8(on0)
  [clr1] -> on_status/7(clr1)
  [clr0] -> on_status/6(clr0)
  ch_split/2(per1) -> config_regs1/1(per)
  config_regs1/4(pd_on) -> [on1]
  config_regs1/3(alarm_clr) -> [clr1]
  config_regs1/2(pk_lim) -> [pk1]
  config_regs0/4(pd_on) -> [on0]
  add_switch/2(y) -> y/1
  on_status/4(sw1) -> [sw1]
  on_status/3(sw0) -> [sw0]
  detect_q/3(sr_alarm) -> on_status/5(srq_alarm)
  detect_q/2(pk_alarm) -> on_status/4(pkq_alarm)
  detect_i/3(sr_alarm) -> on_status/3(sri_alarm)
  detect_i/2(pk_alarm) -> on_status/2(pki_alarm)
  detect_i/1(cho) -> on_status/1(chi)
  Demux2/2 -> detect_q/3(d)
  Demux1/2 -> detect_q/2(x)
  [sr1] -> detect_q/7(sr1)
  [sr0] -> detect_q/6(sr0)
  [pk1] -> detect_q/5(pk1)
  [pk0] -> detect_q/4(pk0)
  [sr1] -> detect_i/7(sr1)
  [sr0] -> detect_i/6(sr0)
  [pk1] -> detect_i/5(pk1)
  [pk0] -> detect_i/4(pk0)
  chi/1 -> detect_i/1(chi), detect_q/1(chi), add_switch/1(chi)
  config_regs0/2(pk_lim) -> [pk0]
  config_regs0/1(sr_lim) -> [sr0]
  Demux2/1 -> detect_i/3(d)
  Demux1/1 -> detect_i/2(x)
  d/1 -> Demux2/1, add_switch/3(d)
  x/1 -> Demux1/1, add_switch/2(x)
  ch_split/1(per0) -> config_regs0/1(per)
  chnsel/1 -> ch_split/2(chnsel), on_status/10(chnsel)
  perbus/1 -> ch_split/1(per)

== system pd_path_sg/resamp_mod ==
  rst : Inport
  chn : Inport  Port=2
  Ai : Inport  Port=3
  Aq : Inport  Port=4
  Bi : Inport  Port=5
  Bq : Inport  Port=6
  LO1 : Subsystem  mask{FTW=115}
  mod0 : Subsystem
  mod1 : Subsystem
  output_samp_E2_p0 : Subsystem
  output_samp_E2_p1 : Subsystem
  output_samp_E2_p2 : Subsystem
  output_samp_E2_p3 : Subsystem
  Ai0 : Outport
  Aq0 : Outport  Port=2
  Ai1 : Outport  Port=3
  Aq1 : Outport  Port=4
  wires:
  Ai/1 -> output_samp_E2_p0/1(Ai)
  Aq/1 -> output_samp_E2_p1/1(Ai)
  Bi/1 -> output_samp_E2_p2/1(Ai)
  Bq/1 -> output_samp_E2_p3/1(Ai)
  chn/1 -> output_samp_E2_p3/2(chn), output_samp_E2_p2/2(chn), output_samp_E2_p1/2(chn), output_samp_E2_p0/2(chn)
  rst/1 -> LO1/1(rst)
  mod0/1(Yi) -> Ai0/1
  mod0/2(Yq) -> Aq0/1
  LO1/1(sin) -> mod1/5(sin), mod0/5(sin)
  LO1/2(cos) -> mod1/6(cos), mod0/6(cos)
  mod1/1(Yi) -> Ai1/1
  mod1/2(Yq) -> Aq1/1
  [low_i0] -> mod0/3(Bi)
  [low_q0] -> mod0/4(Bq)
  [high_i0] -> mod0/1(Ai)
  [high_q0] -> mod0/2(Aq)
  [high_i1] -> mod1/1(Ai)
  [high_q1] -> mod1/2(Aq)
  [low_i1] -> mod1/3(Bi)
  [low_q1] -> mod1/4(Bq)
  output_samp_E2_p0/1(Ai0) -> [low_i0]
  output_samp_E2_p1/1(Ai0) -> [low_q0]
  output_samp_E2_p0/2(Ai1) -> [low_i1]
  output_samp_E2_p1/2(Ai1) -> [low_q1]
  output_samp_E2_p2/1(Ai0) -> [high_i0]
  output_samp_E2_p2/2(Ai1) -> [high_i1]
  output_samp_E2_p3/1(Ai0) -> [high_q0]
  output_samp_E2_p3/2(Ai1) -> [high_q1]

== system pd_path_sg/A_dispatch/config_regs ==
  per : Inport
  Bus Selector : BusSelector  OutputSignals=addr,din,we
  perbus_reg : Subsystem  mask{reg_addr=reg_dltap(para_band+1) + 0}
  perbus_reg1 : Subsystem  mask{reg_addr=reg_dltap(para_band+1) + 1}
  perbus_reg2 : Subsystem  mask{reg_addr=reg_dltap(para_band+1) + 2}
  perbus_reg3 : Subsystem  mask{reg_addr=reg_dltap(para_band+1) + 3}
  perbus_reg4 : Subsystem  mask{reg_addr=reg_dltap(para_band+1) + 4}
  perbus_reg5 : Subsystem  mask{reg_addr=reg_dltap(para_band+1) + 5}
  perbus_reg6 : Subsystem  mask{reg_addr=reg_dltap(para_band+1) + 6}
  dn0 : Outport
  dn1 : Outport  Port=2
  dn2 : Outport  Port=3
  dn3 : Outport  Port=4
  dn4 : Outport  Port=5
  dn5 : Outport  Port=6
  dn6 : Outport  Port=7
  wires:
  perbus_reg6/1(q) -> dn6/1
  perbus_reg5/1(q) -> dn5/1
  perbus_reg4/1(q) -> dn4/1
  perbus_reg3/1(q) -> dn3/1
  perbus_reg2/1(q) -> dn2/1
  perbus_reg1/1(q) -> dn1/1
  perbus_reg/1(q) -> dn0/1
  Bus Selector/1 -> perbus_reg/1(addr), perbus_reg1/1(addr), perbus_reg2/1(addr), perbus_reg3/1(addr), perbus_reg4/1(addr), perbus_reg6/1(addr), perbus_reg5/1(addr)  "<addr>"
  Bus Selector/2 -> perbus_reg/2(din), perbus_reg1/2(din), perbus_reg2/2(din), perbus_reg3/2(din), perbus_reg4/2(din), perbus_reg6/2(din), perbus_reg5/2(din)  "<din>"
  Bus Selector/3 -> perbus_reg/3(we), perbus_reg1/3(we), perbus_reg2/3(we), perbus_reg3/3(we), perbus_reg4/3(we), perbus_reg5/3(we), perbus_reg6/3(we)  "<we>"
  per/1 -> Bus Selector/1

== system pd_path_sg/A_dispatch/iq_delay ==
  x : Inport
  Delay : xbsIndex_r4/Delay  rst=off  infoeditControl=Selection of Reset will increase slice count due to use of real FFs and instead of SRLs  en=off  latency=clocks  reg_retiming=off  dbl_ovrd=off  block_type=delay
      settings: infoedit=Hardware notes: A delay line is a chain, each link of which is an SRL16 or SRL32 followed by a flip-flop.
  Delay1 : xbsIndex_r4/Delay  rst=off  infoeditControl=Selection of Reset will increase slice count due to use of real FFs and instead of SRLs  en=off  latency=clocks  reg_retiming=off  dbl_ovrd=off  block_type=delay
      settings: infoedit=Hardware notes: A delay line is a chain, each link of which is an SRL16 or SRL32 followed by a flip-flop.
  Demux : Demux  Outputs=2
  Mux : Mux  Inputs=2
  y : Outport
  wires:
  Delay1/1 -> Mux/2
  Demux/2 -> Delay1/1
  Demux/1 -> Delay/1
  Mux/1 -> y/1
  Delay/1 -> Mux/1
  x/1 -> Demux/1

== system pd_path_sg/A_dispatch/vdelay0 ==
  dn : Inport
  x : Inport  Port=2
  ab : Inport  Port=3
  Mux : Mux  Inputs=2
  Reinterpret : xbsIndex_r4/Reinterpret  force_arith_type=on  arith_type="Signed  (2's comp)"  force_bin_pt=on  bin_pt=0  block_type=reinterpret
  Reinterpret1 : xbsIndex_r4/Reinterpret  force_arith_type=on  arith_type="Signed  (2's comp)"  force_bin_pt=on  bin_pt=0  block_type=reinterpret
  Slice : xbsIndex_r4/Slice  nbits=6  boolean_output=off  mode=Lower Bit Location + Width  bit1=0  base1=MSB of Input  bit0=0  base0=LSB of Input  dbl_ovrd=off  block_type=slice
  Slice1 : xbsIndex_r4/Slice  nbits=6  boolean_output=off  mode=Lower Bit Location + Width  bit1=0  base1=MSB of Input  bit0=8  base0=LSB of Input  dbl_ovrd=off  block_type=slice
  Slice2 : xbsIndex_r4/Slice  nbits=16  boolean_output=off  mode=Lower Bit Location + Width  bit1=0  base1=MSB of Input  bit0=16  base0=LSB of Input  dbl_ovrd=off  block_type=slice
  Slice3 : xbsIndex_r4/Slice  nbits=16  boolean_output=off  mode=Lower Bit Location + Width  bit1=0  base1=MSB of Input  bit0=0  base0=LSB of Input  dbl_ovrd=off  block_type=slice
  Slice4 : xbsIndex_r4/Slice  nbits=10  boolean_output=off  mode=Lower Bit Location + Width  bit1=0  base1=MSB of Input  bit0=10  base0=LSB of Input  dbl_ovrd=off  block_type=slice
  Slice5 : xbsIndex_r4/Slice  nbits=10  boolean_output=off  mode=Lower Bit Location + Width  bit1=0  base1=MSB of Input  bit0=0  base0=LSB of Input  dbl_ovrd=off  block_type=slice
  asr0 : xbsIndex_r4/Addressable Shift Register  infer_latency=on  depth=64  initVector=[0]  en=off  use_behavioral_HDL=off  Optimization=Resource  dbl_ovrd=off  block_type=addrsr
      settings: infoedit="Delay of configurable length.  Any element in the delay line can be addressed and driven onto the output port.<br><br>Hardware notes: Generates fast, compact FIFO-style shift registers or delay lines using SRL16/SRL32 mode of the slice LUTs"
  asr1 : xbsIndex_r4/Addressable Shift Register  infer_latency=on  depth=64  initVector=[0]  en=off  use_behavioral_HDL=off  Optimization=Resource  dbl_ovrd=off  block_type=addrsr
      settings: infoedit="Delay of configurable length.  Any element in the delay line can be addressed and driven onto the output port.<br><br>Hardware notes: Generates fast, compact FIFO-style shift registers or delay lines using SRL16/SRL32 mode of the slice LUTs"
  regsp : xbsIndex_r4/Delay  rst=off  infoeditControl=Selection of Reset will increase slice count due to use of real FFs and instead of SRLs  en=off  latency=1  reg_retiming=off  dbl_ovrd=off  block_type=delay
      settings: infoedit=Hardware notes: A delay line is a chain, each link of which is an SRL16 or SRL32 followed by a flip-flop.
  regsp1 : xbsIndex_r4/Delay  rst=off  infoeditControl=Selection of Reset will increase slice count due to use of real FFs and instead of SRLs  en=off  latency=1  reg_retiming=off  dbl_ovrd=off  block_type=delay
      settings: infoedit=Hardware notes: A delay line is a chain, each link of which is an SRL16 or SRL32 followed by a flip-flop.
  y : Outport
  ar : Outport  Port=2
  br : Outport  Port=3
  wires:
  Reinterpret1/1 -> Mux/2
  Reinterpret/1 -> Mux/1
  Mux/1 -> y/1
  Slice3/1 -> Reinterpret1/1
  Slice2/1 -> Reinterpret/1
  dn/1 -> Slice/1, Slice1/1
  Slice5/1 -> br/1
  Slice4/1 -> ar/1
  asr1/1 -> regsp1/1
  asr0/1 -> regsp/1
  x/1 -> asr0/1
  Slice/1 -> asr0/2
  ab/1 -> asr1/1
  Slice1/1 -> asr1/2
  regsp/1 -> Slice2/1, Slice3/1
  regsp1/1 -> Slice5/1, Slice4/1
